simulink model "untitled"  (R2019a)
settings: Solver=VariableStepAuto  StartTime=0.0  StopTime=1  RelTol=1e-3
values from neighbouring files (symbols this model uses):
  Ts_Control = 5.0000e-05    (= 5e-05)    [Sec_Impedance.m]
  Ts_Power = 5.0000e-05    (= 5e-05)    [Sec_Impedance.m]
undefined symbols (not defined in the file or in its folder): D1, Delta, Ion, Lithium
libraries: powerlib x152, powerlib_meascontrol x65, simulink x14, electricdrivelib x12, simulink_extras x12
(part 5 of 5)

== system untitled/1MVA Smart EV chargers lot/200-kW 440-V(LN) 3-PH EV Charger/Subsystem ==
  phase shift (-90,90) : Inport
  Add : Sum
  Clock : Clock
  Clock1 : Clock
  Constant2 : Constant  Commented=on  Value=90
  Constant3 : Constant  Value=2*pi*10000
  Constant4 : Constant  Value=2*pi*10000
  Degrees to Radians : simulink_extras/Transformations/Degrees to Radians
  Divide : Product  Inputs=**
  Divide1 : Product  Inputs=**
  Saturation : Saturate  UpperLimit=90  LowerLimit=-90
  Sin : Trigonometry
  Sin1 : Trigonometry
  Uref_DAB1 : Outport
  Uref_DAB2 : Outport  Port=2
  wires:
  Divide1/1 -> Sin1/1
  Divide/1 -> Add/2
  Constant4/1 -> Divide1/1
  Add/1 -> Sin/1
  Saturation/1 -> Degrees to Radians/1
  Degrees to Radians/1 -> Add/1
  Clock1/1 -> Divide1/2
  Clock/1 -> Divide/2
  Constant3/1 -> Divide/1
  Sin/1 -> Uref_DAB2/1  "Uref_DAB2"
  Sin1/1 -> Uref_DAB1/1  "Uref_DAB1"
  phase shift (-90,90)/1 -> Saturation/1

== system untitled/1MVA Smart EV chargers lot/200-kW 440-V(LN) 3-PH EV Charger2/Subsystem ==
  phase shift (-90,90) : Inport
  Add : Sum
  Clock : Clock
  Clock1 : Clock
  Constant2 : Constant  Commented=on  Value=90
  Constant3 : Constant  Value=2*pi*10000
  Constant4 : Constant  Value=2*pi*10000
  Degrees to Radians : simulink_extras/Transformations/Degrees to Radians
  Divide : Product  Inputs=**
  Divide1 : Product  Inputs=**
  Saturation : Saturate  UpperLimit=90  LowerLimit=-90
  Sin : Trigonometry
  Sin1 : Trigonometry
  Uref_DAB1 : Outport
  Uref_DAB2 : Outport  Port=2
  wires:
  Divide1/1 -> Sin1/1
  Divide/1 -> Add/2
  Constant4/1 -> Divide1/1
  Add/1 -> Sin/1
  Saturation/1 -> Degrees to Radians/1
  Degrees to Radians/1 -> Add/1
  Clock1/1 -> Divide1/2
  Clock/1 -> Divide/2
  Constant3/1 -> Divide/1
  Sin/1 -> Uref_DAB2/1  "Uref_DAB2"
  Sin1/1 -> Uref_DAB1/1  "Uref_DAB1"
  phase shift (-90,90)/1 -> Saturation/1

== system untitled/1MVA Smart EV chargers lot/200-kW 440-V(LN) 3-PH EV Charger3/Subsystem ==
  phase shift (-90,90) : Inport
  Add : Sum
  Clock : Clock
  Clock1 : Clock
  Constant2 : Constant  Commented=on  Value=90
  Constant3 : Constant  Value=2*pi*10000
  Constant4 : Constant  Value=2*pi*10000
  Degrees to Radians : simulink_extras/Transformations/Degrees to Radians
  Divide : Product  Inputs=**
  Divide1 : Product  Inputs=**
  Saturation : Saturate  UpperLimit=90  LowerLimit=-90
  Sin : Trigonometry
  Sin1 : Trigonometry
  Uref_DAB1 : Outport
  Uref_DAB2 : Outport  Port=2
  wires:
  Divide1/1 -> Sin1/1
  Divide/1 -> Add/2
  Constant4/1 -> Divide1/1
  Add/1 -> Sin/1
  Saturation/1 -> Degrees to Radians/1
  Degrees to Radians/1 -> Add/1
  Clock1/1 -> Divide1/2
  Clock/1 -> Divide/2
  Constant3/1 -> Divide/1
  Sin/1 -> Uref_DAB2/1  "Uref_DAB2"
  Sin1/1 -> Uref_DAB1/1  "Uref_DAB1"
  phase shift (-90,90)/1 -> Saturation/1

== system untitled/1MVA Smart EV chargers lot/200-kW 440-V(LN) 3-PH EV Charger4/Subsystem ==
  phase shift (-90,90) : Inport
  Add : Sum
  Clock : Clock
  Clock1 : Clock
  Constant2 : Constant  Commented=on  Value=90
  Constant3 : Constant  Value=2*pi*10000
  Constant4 : Constant  Value=2*pi*10000
  Degrees to Radians : simulink_extras/Transformations/Degrees to Radians
  Divide : Product  Inputs=**
  Divide1 : Product  Inputs=**
  Saturation : Saturate  UpperLimit=90  LowerLimit=-90
  Sin : Trigonometry
  Sin1 : Trigonometry
  Uref_DAB1 : Outport
  Uref_DAB2 : Outport  Port=2
  wires:
  Divide1/1 -> Sin1/1
  Divide/1 -> Add/2
  Constant4/1 -> Divide1/1
  Add/1 -> Sin/1
  Saturation/1 -> Degrees to Radians/1
  Degrees to Radians/1 -> Add/1
  Clock1/1 -> Divide1/2
  Clock/1 -> Divide/2
  Constant3/1 -> Divide/1
  Sin/1 -> Uref_DAB2/1  "Uref_DAB2"
  Sin1/1 -> Uref_DAB1/1  "Uref_DAB1"
  phase shift (-90,90)/1 -> Saturation/1

== system untitled/1MVA Smart EV chargers lot/200-kW 440-V(LN) 3-PH EV Charger5/Subsystem ==
  phase shift (-90,90) : Inport
  Add : Sum
  Clock : Clock
  Clock1 : Clock
  Constant2 : Constant  Commented=on  Value=90
  Constant3 : Constant  Value=2*pi*10000
  Constant4 : Constant  Value=2*pi*10000
  Degrees to Radians : simulink_extras/Transformations/Degrees to Radians
  Divide : Product  Inputs=**
  Divide1 : Product  Inputs=**
  Saturation : Saturate  UpperLimit=90  LowerLimit=-90
  Sin : Trigonometry
  Sin1 : Trigonometry
  Uref_DAB1 : Outport
  Uref_DAB2 : Outport  Port=2
  wires:
  Divide1/1 -> Sin1/1
  Divide/1 -> Add/2
  Constant4/1 -> Divide1/1
  Add/1 -> Sin/1
  Saturation/1 -> Degrees to Radians/1
  Degrees to Radians/1 -> Add/1
  Clock1/1 -> Divide1/2
  Clock/1 -> Divide/2
  Constant3/1 -> Divide/1
  Sin/1 -> Uref_DAB2/1  "Uref_DAB2"
  Sin1/1 -> Uref_DAB1/1  "Uref_DAB1"
  phase shift (-90,90)/1 -> Saturation/1

== system untitled/OFF-BOARD EV CHARGER/Subsystem/DQ to Alpha beta ==
  dq0 : Inport  PortDimensions=3
  wt1 : Inport  Port=2  PortDimensions=1
  Demux4 : Demux  Outputs=[2 1]
  Fcn : Fcn  Expr=u[1]*sin(u[3]) + u[2]*cos(u[3])
  Fcn1 : Fcn  Expr=-u[1]*cos(u[3]) + u[2]*sin(u[3])
  Mux1 : Mux  Inputs=[2 1]
  Mux4 : Mux  Inputs=2
  Mux5 : Mux  Inputs=[2 1]
  Mux6 : Mux  Inputs=[2 1]
  al_be_0 : Outport
  wires:
  Mux4/1 -> Mux1/1
  Mux6/1 -> Fcn1/1
  Fcn1/1 -> Mux4/2
  Demux4/1 -> Mux6/1, Mux5/1
  Mux5/1 -> Fcn/1
  Demux4/2 -> Mux1/2
  Fcn/1 -> Mux4/1
  wt1/1 -> Mux5/2, Mux6/2
  dq0/1 -> Demux4/1
  Mux1/1 -> al_be_0/1

== system untitled/OFF-BOARD EV CHARGER/Subsystem1/Subsystem1 ==
  note: q = al*cos(wt) + be*sin(wt)
  note: d = al*sin(wt) - be*cos(wt)
  al_be : Inport  PortDimensions=2
  wt1 : Inport  Port=2  PortDimensions=1
  Fcn : Fcn  Expr=u[1]*sin(u[3]) - u[2]*cos(u[3])
  Fcn1 : Fcn  Expr=u[1]*cos(u[3]) + u[2]*sin(u[3])
  Mux4 : Mux  Inputs=2
  Mux5 : Mux  Inputs=[2 1]
  Mux6 : Mux  Inputs=[2 1]
  dq : Outport
  wires:
  Mux5/1 -> Fcn/1
  Fcn1/1 -> Mux4/2
  al_be/1 -> Mux6/1, Mux5/1
  wt1/1 -> Mux5/2, Mux6/2
  Mux6/1 -> Fcn1/1
  Fcn/1 -> Mux4/1
  Mux4/1 -> dq/1

== system untitled/OFF-BOARD EV CHARGER/Subsystem2/Subsystem1 ==
  note: q = al*cos(wt) + be*sin(wt)
  note: d = al*sin(wt) - be*cos(wt)
  al_be : Inport  PortDimensions=2
  wt1 : Inport  Port=2  PortDimensions=1
  Fcn : Fcn  Expr=u[1]*sin(u[3]) - u[2]*cos(u[3])
  Fcn1 : Fcn  Expr=u[1]*cos(u[3]) + u[2]*sin(u[3])
  Mux4 : Mux  Inputs=2
  Mux5 : Mux  Inputs=[2 1]
  Mux6 : Mux  Inputs=[2 1]
  dq : Outport
  wires:
  Mux5/1 -> Fcn/1
  Fcn1/1 -> Mux4/2
  al_be/1 -> Mux6/1, Mux5/1
  wt1/1 -> Mux5/2, Mux6/2
  Mux6/1 -> Fcn1/1
  Fcn/1 -> Mux4/1
  Mux4/1 -> dq/1

== system untitled/OFF-BOARD EV CHARGER1/Subsystem/DQ to Alpha beta ==
  dq0 : Inport  PortDimensions=3
  wt1 : Inport  Port=2  PortDimensions=1
  Demux4 : Demux  Outputs=[2 1]
  Fcn : Fcn  Expr=u[1]*sin(u[3]) + u[2]*cos(u[3])
  Fcn1 : Fcn  Expr=-u[1]*cos(u[3]) + u[2]*sin(u[3])
  Mux1 : Mux  Inputs=[2 1]
  Mux4 : Mux  Inputs=2
  Mux5 : Mux  Inputs=[2 1]
  Mux6 : Mux  Inputs=[2 1]
  al_be_0 : Outport
  wires:
  Mux4/1 -> Mux1/1
  Mux6/1 -> Fcn1/1
  Fcn1/1 -> Mux4/2
  Demux4/1 -> Mux6/1, Mux5/1
  Mux5/1 -> Fcn/1
  Demux4/2 -> Mux1/2
  Fcn/1 -> Mux4/1
  wt1/1 -> Mux5/2, Mux6/2
  dq0/1 -> Demux4/1
  Mux1/1 -> al_be_0/1

== system untitled/OFF-BOARD EV CHARGER1/Subsystem1/Subsystem1 ==
  note: q = al*cos(wt) + be*sin(wt)
  note: d = al*sin(wt) - be*cos(wt)
  al_be : Inport  PortDimensions=2
  wt1 : Inport  Port=2  PortDimensions=1
  Fcn : Fcn  Expr=u[1]*sin(u[3]) - u[2]*cos(u[3])
  Fcn1 : Fcn  Expr=u[1]*cos(u[3]) + u[2]*sin(u[3])
  Mux4 : Mux  Inputs=2
  Mux5 : Mux  Inputs=[2 1]
  Mux6 : Mux  Inputs=[2 1]
  dq : Outport
  wires:
  Mux5/1 -> Fcn/1
  Fcn1/1 -> Mux4/2
  al_be/1 -> Mux6/1, Mux5/1
  wt1/1 -> Mux5/2, Mux6/2
  Mux6/1 -> Fcn1/1
  Fcn/1 -> Mux4/1
  Mux4/1 -> dq/1

== system untitled/OFF-BOARD EV CHARGER1/Subsystem2/Subsystem1 ==
  note: q = al*cos(wt) + be*sin(wt)
  note: d = al*sin(wt) - be*cos(wt)
  al_be : Inport  PortDimensions=2
  wt1 : Inport  Port=2  PortDimensions=1
  Fcn : Fcn  Expr=u[1]*sin(u[3]) - u[2]*cos(u[3])
  Fcn1 : Fcn  Expr=u[1]*cos(u[3]) + u[2]*sin(u[3])
  Mux4 : Mux  Inputs=2
  Mux5 : Mux  Inputs=[2 1]
  Mux6 : Mux  Inputs=[2 1]
  dq : Outport
  wires:
  Mux5/1 -> Fcn/1
  Fcn1/1 -> Mux4/2
  al_be/1 -> Mux6/1, Mux5/1
  wt1/1 -> Mux5/2, Mux6/2
  Mux6/1 -> Fcn1/1
  Fcn/1 -> Mux4/1
  Mux4/1 -> dq/1

== system untitled/OFF-BOARD EV CHARGER2/Subsystem/DQ to Alpha beta ==
  dq0 : Inport  PortDimensions=3
  wt1 : Inport  Port=2  PortDimensions=1
  Demux4 : Demux  Outputs=[2 1]
  Fcn : Fcn  Expr=u[1]*sin(u[3]) + u[2]*cos(u[3])
  Fcn1 : Fcn  Expr=-u[1]*cos(u[3]) + u[2]*sin(u[3])
  Mux1 : Mux  Inputs=[2 1]
  Mux4 : Mux  Inputs=2
  Mux5 : Mux  Inputs=[2 1]
  Mux6 : Mux  Inputs=[2 1]
  al_be_0 : Outport
  wires:
  Mux4/1 -> Mux1/1
  Mux6/1 -> Fcn1/1
  Fcn1/1 -> Mux4/2
  Demux4/1 -> Mux6/1, Mux5/1
  Mux5/1 -> Fcn/1
  Demux4/2 -> Mux1/2
  Fcn/1 -> Mux4/1
  wt1/1 -> Mux5/2, Mux6/2
  dq0/1 -> Demux4/1
  Mux1/1 -> al_be_0/1

== system untitled/OFF-BOARD EV CHARGER2/Subsystem1/Subsystem1 ==
  note: q = al*cos(wt) + be*sin(wt)
  note: d = al*sin(wt) - be*cos(wt)
  al_be : Inport  PortDimensions=2
  wt1 : Inport  Port=2  PortDimensions=1
  Fcn : Fcn  Expr=u[1]*sin(u[3]) - u[2]*cos(u[3])
  Fcn1 : Fcn  Expr=u[1]*cos(u[3]) + u[2]*sin(u[3])
  Mux4 : Mux  Inputs=2
  Mux5 : Mux  Inputs=[2 1]
  Mux6 : Mux  Inputs=[2 1]
  dq : Outport
  wires:
  Mux5/1 -> Fcn/1
  Fcn1/1 -> Mux4/2
  al_be/1 -> Mux6/1, Mux5/1
  wt1/1 -> Mux5/2, Mux6/2
  Mux6/1 -> Fcn1/1
  Fcn/1 -> Mux4/1
  Mux4/1 -> dq/1

== system untitled/OFF-BOARD EV CHARGER2/Subsystem2/Subsystem1 ==
  note: q = al*cos(wt) + be*sin(wt)
  note: d = al*sin(wt) - be*cos(wt)
  al_be : Inport  PortDimensions=2
  wt1 : Inport  Port=2  PortDimensions=1
  Fcn : Fcn  Expr=u[1]*sin(u[3]) - u[2]*cos(u[3])
  Fcn1 : Fcn  Expr=u[1]*cos(u[3]) + u[2]*sin(u[3])
  Mux4 : Mux  Inputs=2
  Mux5 : Mux  Inputs=[2 1]
  Mux6 : Mux  Inputs=[2 1]
  dq : Outport
  wires:
  Mux5/1 -> Fcn/1
  Fcn1/1 -> Mux4/2
  al_be/1 -> Mux6/1, Mux5/1
  wt1/1 -> Mux5/2, Mux6/2
  Mux6/1 -> Fcn1/1
  Fcn/1 -> Mux4/1
  Mux4/1 -> dq/1

== system untitled/OFF-BOARD EV CHARGER3/Subsystem/DQ to Alpha beta ==
  dq0 : Inport  PortDimensions=3
  wt1 : Inport  Port=2  PortDimensions=1
  Demux4 : Demux  Outputs=[2 1]
  Fcn : Fcn  Expr=u[1]*sin(u[3]) + u[2]*cos(u[3])
  Fcn1 : Fcn  Expr=-u[1]*cos(u[3]) + u[2]*sin(u[3])
  Mux1 : Mux  Inputs=[2 1]
  Mux4 : Mux  Inputs=2
  Mux5 : Mux  Inputs=[2 1]
  Mux6 : Mux  Inputs=[2 1]
  al_be_0 : Outport
  wires:
  Mux4/1 -> Mux1/1
  Mux6/1 -> Fcn1/1
  Fcn1/1 -> Mux4/2
  Demux4/1 -> Mux6/1, Mux5/1
  Mux5/1 -> Fcn/1
  Demux4/2 -> Mux1/2
  Fcn/1 -> Mux4/1
  wt1/1 -> Mux5/2, Mux6/2
  dq0/1 -> Demux4/1
  Mux1/1 -> al_be_0/1

== system untitled/OFF-BOARD EV CHARGER3/Subsystem1/Subsystem1 ==
  note: q = al*cos(wt) + be*sin(wt)
  note: d = al*sin(wt) - be*cos(wt)
  al_be : Inport  PortDimensions=2
  wt1 : Inport  Port=2  PortDimensions=1
  Fcn : Fcn  Expr=u[1]*sin(u[3]) - u[2]*cos(u[3])
  Fcn1 : Fcn  Expr=u[1]*cos(u[3]) + u[2]*sin(u[3])
  Mux4 : Mux  Inputs=2
  Mux5 : Mux  Inputs=[2 1]
  Mux6 : Mux  Inputs=[2 1]
  dq : Outport
  wires:
  Mux5/1 -> Fcn/1
  Fcn1/1 -> Mux4/2
  al_be/1 -> Mux6/1, Mux5/1
  wt1/1 -> Mux5/2, Mux6/2
  Mux6/1 -> Fcn1/1
  Fcn/1 -> Mux4/1
  Mux4/1 -> dq/1

== system untitled/OFF-BOARD EV CHARGER3/Subsystem2/Subsystem1 ==
  note: q = al*cos(wt) + be*sin(wt)
  note: d = al*sin(wt) - be*cos(wt)
  al_be : Inport  PortDimensions=2
  wt1 : Inport  Port=2  PortDimensions=1
  Fcn : Fcn  Expr=u[1]*sin(u[3]) - u[2]*cos(u[3])
  Fcn1 : Fcn  Expr=u[1]*cos(u[3]) + u[2]*sin(u[3])
  Mux4 : Mux  Inputs=2
  Mux5 : Mux  Inputs=[2 1]
  Mux6 : Mux  Inputs=[2 1]
  dq : Outport
  wires:
  Mux5/1 -> Fcn/1
  Fcn1/1 -> Mux4/2
  al_be/1 -> Mux6/1, Mux5/1
  wt1/1 -> Mux5/2, Mux6/2
  Mux6/1 -> Fcn1/1
  Fcn/1 -> Mux4/1
  Mux4/1 -> dq/1

== system untitled/OFF-BOARD EV CHARGER4/Subsystem/DQ to Alpha beta ==
  dq0 : Inport  PortDimensions=3
  wt1 : Inport  Port=2  PortDimensions=1
  Demux4 : Demux  Outputs=[2 1]
  Fcn : Fcn  Expr=u[1]*sin(u[3]) + u[2]*cos(u[3])
  Fcn1 : Fcn  Expr=-u[1]*cos(u[3]) + u[2]*sin(u[3])
  Mux1 : Mux  Inputs=[2 1]
  Mux4 : Mux  Inputs=2
  Mux5 : Mux  Inputs=[2 1]
  Mux6 : Mux  Inputs=[2 1]
  al_be_0 : Outport
  wires:
  Mux4/1 -> Mux1/1
  Mux6/1 -> Fcn1/1
  Fcn1/1 -> Mux4/2
  Demux4/1 -> Mux6/1, Mux5/1
  Mux5/1 -> Fcn/1
  Demux4/2 -> Mux1/2
  Fcn/1 -> Mux4/1
  wt1/1 -> Mux5/2, Mux6/2
  dq0/1 -> Demux4/1
  Mux1/1 -> al_be_0/1

== system untitled/OFF-BOARD EV CHARGER4/Subsystem1/Subsystem1 ==
  note: q = al*cos(wt) + be*sin(wt)
  note: d = al*sin(wt) - be*cos(wt)
  al_be : Inport  PortDimensions=2
  wt1 : Inport  Port=2  PortDimensions=1
  Fcn : Fcn  Expr=u[1]*sin(u[3]) - u[2]*cos(u[3])
  Fcn1 : Fcn  Expr=u[1]*cos(u[3]) + u[2]*sin(u[3])
  Mux4 : Mux  Inputs=2
  Mux5 : Mux  Inputs=[2 1]
  Mux6 : Mux  Inputs=[2 1]
  dq : Outport
  wires:
  Mux5/1 -> Fcn/1
  Fcn1/1 -> Mux4/2
  al_be/1 -> Mux6/1, Mux5/1
  wt1/1 -> Mux5/2, Mux6/2
  Mux6/1 -> Fcn1/1
  Fcn/1 -> Mux4/1
  Mux4/1 -> dq/1

== system untitled/OFF-BOARD EV CHARGER4/Subsystem2/Subsystem1 ==
  note: q = al*cos(wt) + be*sin(wt)
  note: d = al*sin(wt) - be*cos(wt)
  al_be : Inport  PortDimensions=2
  wt1 : Inport  Port=2  PortDimensions=1
  Fcn : Fcn  Expr=u[1]*sin(u[3]) - u[2]*cos(u[3])
  Fcn1 : Fcn  Expr=u[1]*cos(u[3]) + u[2]*sin(u[3])
  Mux4 : Mux  Inputs=2
  Mux5 : Mux  Inputs=[2 1]
  Mux6 : Mux  Inputs=[2 1]
  dq : Outport
  wires:
  Mux5/1 -> Fcn/1
  Fcn1/1 -> Mux4/2
  al_be/1 -> Mux6/1, Mux5/1
  wt1/1 -> Mux5/2, Mux6/2
  Mux6/1 -> Fcn1/1
  Fcn/1 -> Mux4/1
  Mux4/1 -> dq/1

== matlab function untitled/1MVA Smart EV chargers lot/200-kW 440-V(LN) 3-PH EV Charger2/MATLAB Function ==
  data: P input; id output; Q input; vd input; iq output
function [id, iq]= fcn(P, Q, vd)

id = (2*P)/(3*vd);
iq = -(2*Q)/(3*vd);

== matlab function untitled/1MVA Smart EV chargers lot/200-kW 440-V(LN) 3-PH EV Charger/MATLAB Function ==
  data: P input; id output; Q input; vd input; iq output
function [id, iq]= fcn(P, Q, vd)

id = (2*P)/(3*vd);
iq = -(2*Q)/(3*vd);

== matlab function untitled/1MVA Smart EV chargers lot/200-kW 440-V(LN) 3-PH EV Charger3/MATLAB Function ==
  data: P input; id output; Q input; vd input; iq output
function [id, iq]= fcn(P, Q, vd)

id = (2*P)/(3*vd);
iq = -(2*Q)/(3*vd);

== matlab function untitled/1MVA Smart EV chargers lot/200-kW 440-V(LN) 3-PH EV Charger4/MATLAB Function ==
  data: P input; id output; Q input; vd input; iq output
function [id, iq]= fcn(P, Q, vd)

id = (2*P)/(3*vd);
iq = -(2*Q)/(3*vd);

== matlab function untitled/1MVA Smart EV chargers lot/200-kW 440-V(LN) 3-PH EV Charger5/MATLAB Function ==
  data: P input; id output; Q input; vd input; iq output
function [id, iq]= fcn(P, Q, vd)

id = (2*P)/(3*vd);
iq = -(2*Q)/(3*vd);

== matlab function untitled/1MVA Smart EV chargers lot/MATLAB Function ==
  data: Q output; Qreq input; Qcap_total output; Qcap input
function [Q, Qcap_total]= aggregator(Qreq,Qcap)

%las señales de Qcap estan ordenadas secuencialmente desde el cargador 1 hasta el 5; es
%decir, Qcap(1)=Capacidad cargador 1, y asi sicesivamente. 
   
    
Qcap_total=0;
for i=1: length(Qcap)
    Qcap_total = Qcap_total + Qcap(i);
end

if Qreq >= Qcap_total
    Qreq=Qcap_total;
end

Q=zeros(1,length(Qcap))


for i=1: length(Qcap)
    Q(1,i)=(Qcap(i)/Qcap_total)*Qreq;
end

== matlab function untitled/200-kW 440-V(LN) 3-PH EV Charger5/MATLAB Function ==
  data: P input; id output; Q input; vd input; iq output
function [id, iq]= fcn(P, Q, vd)

id = (2*P)/(3*vd);
iq = -(2*Q)/(3*vd);

== matlab function untitled/MATLAB Function ==
  data: Q output; Qreq input; Qcap_total output; Qcap input
function [Q, Qcap_total]= aggregator(Qreq,Qcap)

%las señales de Qcap estan ordenadas secuencialmente desde el cargador 1 hasta el 5; es
%decir, Qcap(1)=Capacidad cargador 1, y asi sicesivamente. 
   
    
Qcap_total=0;
for i=1: length(Qcap)
    Qcap_total = Qcap_total + Qcap(i);
end

if Qreq >= Qcap_total
    Qreq=Qcap_total;
end

Q=zeros(1,length(Qcap))


for i=1: length(Qcap)
    Q(1,i)=(Qcap(i)/Qcap_total)*Qreq;
end

== matlab function untitled/200-kW 440-V(LN) 3-PH EV Charger2/MATLAB Function ==
  data: P input; id output; Q input; vd input; iq output
function [id, iq]= fcn(P, Q, vd)

id = (2*P)/(3*vd);
iq = -(2*Q)/(3*vd);

== matlab function untitled/OFF-BOARD EV CHARGER/MATLAB Function ==
  data: u input; y1 output; y2 output; y3 output
function [y1, y2, y3] = sine_funtion(u)

y1 = sin(2*pi*60*u);
y2 = sin(2*pi*60*u+2*pi/3);
y3 = sin(2*pi*60*u+4*pi/3);

== matlab function untitled/OFF-BOARD EV CHARGER/MATLAB Function1 ==
  data: P input; id output; Q input; vd input; iq output
function [id, iq]= fcn(P, Q, vd)

id = (2*P)/(3*vd);
iq = -(2*Q)/(3*vd);

== matlab function untitled/OFF-BOARD EV CHARGER1/MATLAB Function ==
  data: u input; y1 output; y2 output; y3 output
function [y1, y2, y3] = sine_funtion(u)

y1 = sin(2*pi*60*u);
y2 = sin(2*pi*60*u+2*pi/3);
y3 = sin(2*pi*60*u+4*pi/3);

== matlab function untitled/OFF-BOARD EV CHARGER1/MATLAB Function1 ==
  data: P input; id output; Q input; vd input; iq output
function [id, iq]= fcn(P, Q, vd)

id = (2*P)/(3*vd);
iq = -(2*Q)/(3*vd);

== matlab function untitled/MATLAB Function1 ==
  data: Q output; Qreq input; Qcap_total output; Qcap input
function [Q, Qcap_total]= aggregator(Qreq,Qcap)

%las señales de Qcap estan ordenadas secuencialmente desde el cargador 1 hasta el 5; es
%decir, Qcap(1)=Capacidad cargador 1, y asi sicesivamente. 
   
    
Qcap_total=0;
for i=1: length(Qcap)
    Qcap_total = Qcap_total + Qcap(i);
end

if Qreq >= Qcap_total
    Qreq=Qcap_total;
end

Q=zeros(1,length(Qcap))


for i=1: length(Qcap)
    Q(i)=(Qcap(i)/Qcap_total)*Qreq;
end

== matlab function untitled/OFF-BOARD EV CHARGER2/MATLAB Function ==
  data: u input; y1 output; y2 output; y3 output
function [y1, y2, y3] = sine_funtion(u)

y1 = sin(2*pi*60*u);
y2 = sin(2*pi*60*u+2*pi/3);
y3 = sin(2*pi*60*u+4*pi/3);

== matlab function untitled/OFF-BOARD EV CHARGER2/MATLAB Function1 ==
  data: P input; id output; Q input; vd input; iq output
function [id, iq]= fcn(P, Q, vd)

id = (2*P)/(3*vd);
iq = -(2*Q)/(3*vd);

== matlab function untitled/OFF-BOARD EV CHARGER3/MATLAB Function ==
  data: u input; y1 output; y2 output; y3 output
function [y1, y2, y3] = sine_funtion(u)

y1 = sin(2*pi*60*u);
y2 = sin(2*pi*60*u+2*pi/3);
y3 = sin(2*pi*60*u+4*pi/3);

== matlab function untitled/OFF-BOARD EV CHARGER3/MATLAB Function1 ==
  data: P input; id output; Q input; vd input; iq output
function [id, iq]= fcn(P, Q, vd)

id = (2*P)/(3*vd);
iq = -(2*Q)/(3*vd);

== matlab function untitled/OFF-BOARD EV CHARGER4/MATLAB Function ==
  data: u input; y1 output; y2 output; y3 output
function [y1, y2, y3] = sine_funtion(u)

y1 = sin(2*pi*60*u);
y2 = sin(2*pi*60*u+2*pi/3);
y3 = sin(2*pi*60*u+4*pi/3);

== matlab function untitled/OFF-BOARD EV CHARGER4/MATLAB Function1 ==
  data: P input; id output; Q input; vd input; iq output
function [id, iq]= fcn(P, Q, vd)

id = (2*P)/(3*vd);
iq = -(2*Q)/(3*vd);
